simulink model "ex4sim"  (R2025b)
settings: Solver=VariableStepAuto  StartTime=0.0  StopTime=10.0  RelTol=1e-3
values from neighbouring files (symbols this model uses):
  C = [1 0]    [ex1.m]    (also in ex2.m = [1 1 0])
undefined symbols (not defined in the file or in its folder): L, R, RC

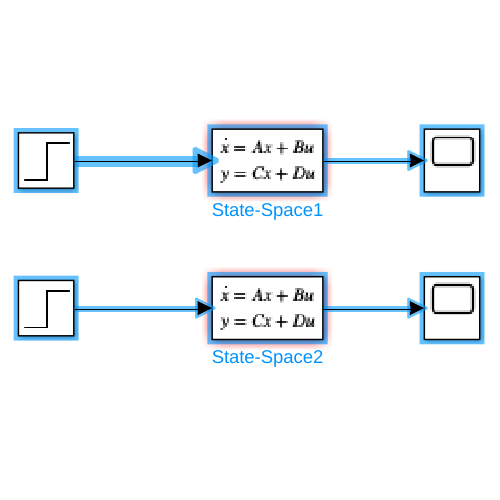
[thumbnail: Simulink's stored preview of the top-level diagram]
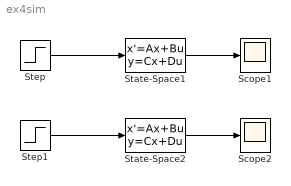
== system ex4sim ==
  Scope1 : Scope
      settings: ActiveDisplayYMinimum=-0.81050635542712857  ActiveDisplayYMaximum=2.7238816183177885
  Scope2 : Scope
      settings: ActiveDisplayYMinimum=-0.81050635542712857  ActiveDisplayYMaximum=2.7238816183177885  DataLoggingVariableName=ScopeData2
  State-Space1 : StateSpace  A=[-RC]  B=[RC]  C=[1]  D=0  InitialCondition=0
  State-Space2 : StateSpace  A=[-R/L, -1/(L*R); 1, 0]  B=[1; 0]  C=[0, 1/(L*C)]  D=0  InitialCondition=0
  Step : Step  SampleTime=0
  Step1 : Step  SampleTime=0
  wires:
  State-Space2/1 -> Scope2/1
  State-Space1/1 -> Scope1/1
  Step1/1 -> State-Space2/1
  Step/1 -> State-Space1/1
